simulink model "CaseMuxTwo"  (R2023b)
settings: Solver=VariableStepAuto  StartTime=0.0  StopTime=10.0  RelTol=1e-3
settings Model: Creator=jsonm  LastModifiedBy=jsonm

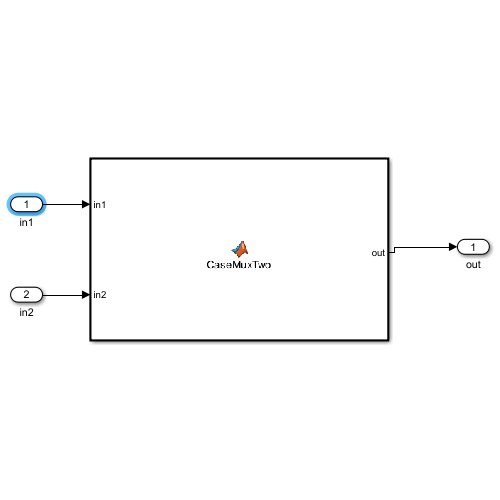
[thumbnail: Simulink's stored preview of the top-level diagram]
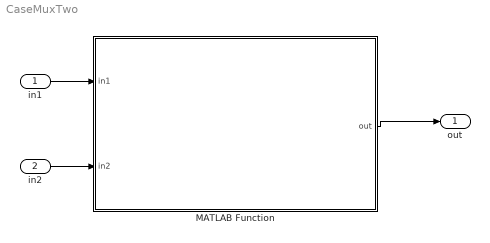
== system CaseMuxTwo ==
  in1 : Inport
  in2 : Inport  Port=2
  MATLAB Function : MATLAB Function  TreatAsAtomicUnit=on
  out : Outport
  wires:
  in1/1 -> MATLAB Function/1(in1)
  in2/1 -> MATLAB Function/2(in2)
  MATLAB Function/1(out) -> out/1

== matlab function CaseMuxTwo/MATLAB Function ==
  data: in1 input; out output; in2 input
function out = CaseMuxTwo(in1, in2)

% Method to mux two inputs into one of two possible outputs based on first
% non-negative input
%
% Written by: Darian Muresan
% Modified by: Jason McCauley

if nargin < 1
    in1 = -1;
    in2 = -1;
elseif nargin < 2
    in2 = -1;
end

if in1 >= 0
    out = in1;
elseif in2 >= 0
    out = in2;
else
    out = -1;
end
